simulink model "forceWithQP"  (Simulink 8.0)
settings: Solver=ode45  StartTime=0.0  StopTime=10.0  RelTol=1e-3
settings Model: Creator=icub  LastModifiedBy=icub

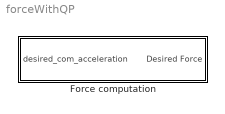
== system forceWithQP ==
  Force computation : Subsystem

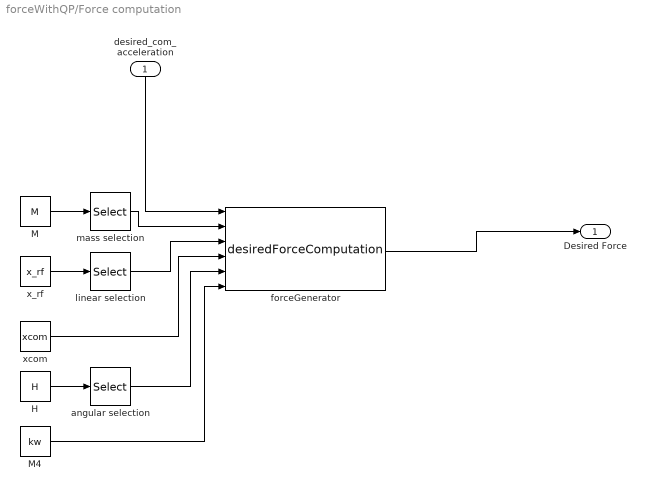
== system forceWithQP/Force computation ==
  desired_com_acceleration : Inport
  H : DataStoreRead  DataStoreName=H
  M : DataStoreRead  DataStoreName=M
  M4 : DataStoreRead  DataStoreName=kw
  angular selection : Selector  InputPortWidth=6  IndexOptions=Index vector (dialog)  Indices=[4:6]  OutputSizes=1
  forceGenerator : M-S-Function  FunctionName=desiredForceComputation
  linear selection : Selector  InputPortWidth=7  IndexOptions=Index vector (dialog)  Indices=[1:3]  OutputSizes=1
  mass selection : Selector  NumberOfDimensions=2  InputPortWidth=3  IndexOptions=Index vector (dialog),Index vector (dialog)  Indices=1,1  OutputSizes=1,1
  x_rf : DataStoreRead  DataStoreName=x_rf
  xcom : DataStoreRead  DataStoreName=xcom
  Desired Force : Outport
  wires:
  mass selection/1 -> forceGenerator/2
  x_rf/1 -> linear selection/1
  xcom/1 -> forceGenerator/4
  desired_com_acceleration/1 -> forceGenerator/1
  M/1 -> mass selection/1
  linear selection/1 -> forceGenerator/3
  angular selection/1 -> forceGenerator/5
  H/1 -> angular selection/1
  M4/1 -> forceGenerator/6
  forceGenerator/1 -> Desired Force/1
